simulink model "robotROSOmnidirectionalFBVisualizationV8_TrayectoriaV2"  (R2020a)
settings: Solver=FixedStepDiscrete  StartTime=0.0  StopTime=inf  FixedStep=0.01  RelTol=1e-3  EnableMultiTasking=on
undefined symbols (not defined in the file): Angular, Linear
libraries: robotlib x4
settings Model: Creator=The MathWorks, Inc.  LastModifiedBy=OsEmm
settings DataIOCC: LimitDataPoints=on  SaveFormat=Array  ReturnWorkspaceOutputs=off
settings OptimizationCC: LifeSpan=Inf  MaxStackSize=64
settings DebuggingCC: SolverPrmCheckMsg=warning  SFUnexpectedBacktrackingDiag=warning  SFNoUnconditionalDefaultTransitionDiag=warning  SFExecutionAtInitializationDiag=none  ArithmeticOperatorsInVariantConditions=warning
settings HardwareCC: ProdBitPerPointer=32  ProdBitPerSizeT=32  ProdBitPerPtrDiffT=32  ProdLargestAtomicFloat=None  ProdIntDivRoundTo=Undefined  ProdEndianess=Unspecified  ProdWordSize=32  ProdHWDeviceType=Generic->Unspecified (assume 32-bit Generic)  UseEmbeddedCoderFeatures=off
settings ModelReferenceCC: PropagateSignalLabelsOutOfModel=off
settings SFSimCC: SimUseLocalCustomCode=off
settings RTWCC: SystemTargetFile=ert.tlc  HardwareBoard=Robot Operating System (ROS)  TLCOptions=-aInlineSetEventsForThisBaseRateFcn=TLC_FALSE -aSuppressMultiTaskScheduler=TLC_FALSE -aRateBasedStepFcn=0  TemplateMakefile=ert_default_tmf  RTWUseLocalCustomCode=off  Toolchain=Catkin  TargetLang=C++
settings CodeAppCC: StateflowObjectComments=on
settings ERTTargetCC: MultiwordLength=2048  ERTCustomFileBanners=off  SupportContinuousTime=on  SupportNonInlinedSFcns=on  RemoveResetFunc=off  SupportVariableSizeSignals=on  ModelStepFunctionPrototypeControlCompliant=off  ConvertIfToSwitch=off  SuppressUnreachableDefaultCases=off
settings ConfigComp: CovMetricSettings=dw  CovHtmlReporting=on  CovSaveCumulativeToWorkspaceVar=on  CovSaveSingleToWorkspaceVar=on  CovExternalEMLEnable=off  CovSFcnEnable=off

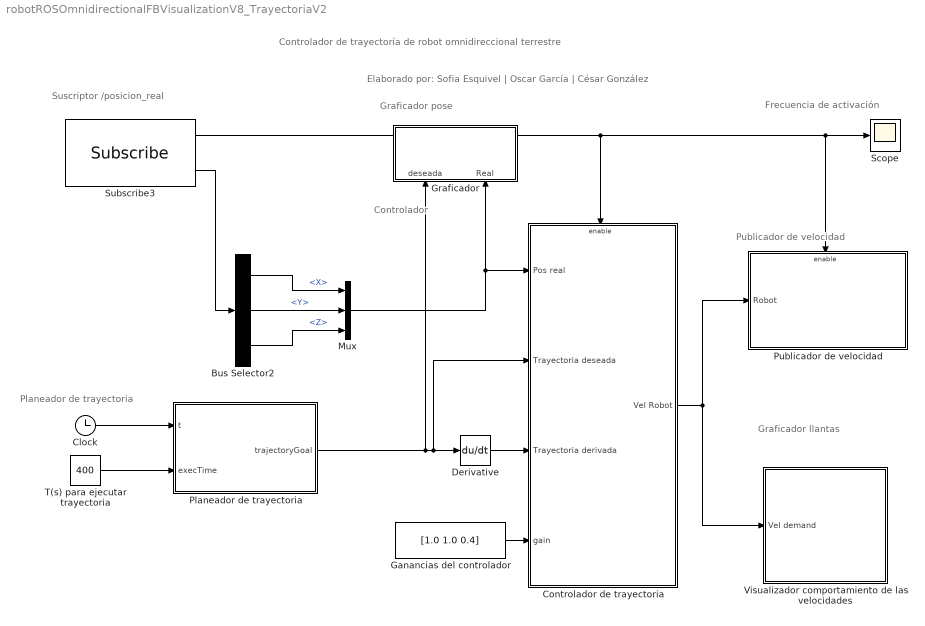
== system robotROSOmnidirectionalFBVisualizationV8_TrayectoriaV2 ==
  note: Frecuencia de activación
  note: Graficador llantas
  note: Publicador de velocidad
  note: Controlador
  note: Planeador de trayectoria
  note: Graficador pose
  note: Suscriptor /posicion_real
  note: Elaborado por: Sofia Esquivel | Oscar García | César González
  note: Controlador de trayectoría de robot omnidireccional terrestre
  Bus Selector2 : BusSelector  DialogController=Simulink.DDGSource_BusSelector  OutputSignals=Position.X,Position.Y,Position.Z
  Clock : Clock
  "Controlador de trayectoria " : Subsystem
  Derivative : Derivative
  Ganancias del controlador : Constant  Value=[1.0 1.0 0.4]
  Graficador : Subsystem
      settings: PortSchema="{\"entries\":[{\"content\":{\"sides\":[{\"content\":{\"connectorIds\":[]},\"type\":\"ConnectorPlacement.EquallySpacedRectSide\",\"uuid\":\"ca5a2c3c-1c6a-4a59-81b5-e28a07e4aa01\"},{\"content\":{\"connectorIds\":[],\"side\":\"RIGHT\"},\"type\":\"ConnectorPlacement.EquallySpacedRectSide\",\"uuid\":\"c66d5d4f-c2ca-4972-b9ac-4479b8aa35e9\"},{\"content\":{\"connectorIds\":[],\"side\":\"TOP\"},\"type\":\"ConnectorPlacement.EquallySpacedRectSide\",\"uuid\":\"6ec84811-9ba3-4605-b969-ad2255866a28\"},{\"content\":{\"connectorIds\":[\"In1\",\"In2\"],\"side\":\"BOTTOM\"},\"type\":\"ConnectorPlacement.EquallySpacedRectSide\",\"uuid\":\"853aacb6-3c5a-4075-8dd4-dac3c2fac177\"}]},\"type\":\"ConnectorPlacement.EquallySpacedConnector\",\"uuid\":\"ad9aaa3d-d9b2-4c1e-8caf-17ebb9e3127a\"}],\"packageUris\":[\"http://schema.mathworks.com/mf0/Connector/19700101\"],\"version\":\"1.0\"}"
  Mux : Mux  Inputs=3
  Planeador de trayectoria : MATLAB Function  TreatAsAtomicUnit=on
  Publicador de velocidad : Subsystem
  Scope : Scope
  Subscribe3 : robotlib/Subscribe  topicSource=Select from ROS network  topic=/posicion_real  messageType=geometry_msgs/Pose  sampleTime=-1  messageQueueLength=51
  "T(s) para ejecutar trayectoria " : Constant  Value=400
  "Visualizador comportamiento de las velocidades " : Subsystem
  wires:
  Subscribe3/1 -> Publicador de velocidad/Enable, Scope/1, "Controlador de trayectoria "/Enable
  Subscribe3/2 -> Bus Selector2/1
  Bus Selector2/1 -> Mux/1  "<X>"
  Bus Selector2/2 -> Mux/2  "<Y>"
  Bus Selector2/3 -> Mux/3  "<Z>"
  Mux/1 -> Graficador/2(Real), "Controlador de trayectoria "/1(Pos real)
  "Controlador de trayectoria "/1(Vel Robot) -> "Visualizador comportamiento de las velocidades "/1(Vel demand), Publicador de velocidad/1(Robot)
  Derivative/1 -> "Controlador de trayectoria "/3("Trayectoria derivada ")
  Clock/1 -> Planeador de trayectoria/1(t)
  "T(s) para ejecutar trayectoria "/1 -> Planeador de trayectoria/2(execTime)
  Planeador de trayectoria/1(trajectoryGoal) -> Graficador/1(deseada), "Controlador de trayectoria "/2(Trayectoria deseada), Derivative/1
  Ganancias del controlador/1 -> "Controlador de trayectoria "/4(gain)

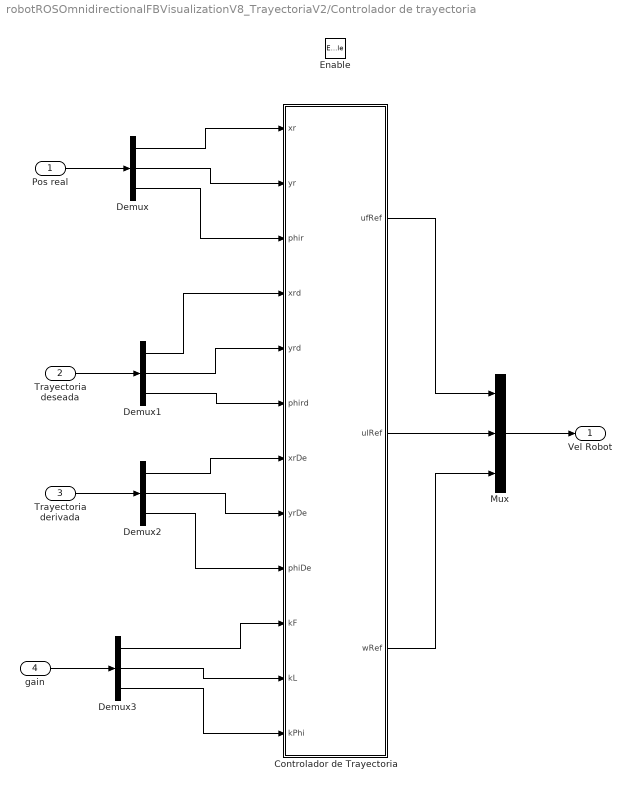
== system robotROSOmnidirectionalFBVisualizationV8_TrayectoriaV2/Controlador de trayectoria  ==
  Pos real : Inport
  Trayectoria deseada : Inport  Port=2
  "Trayectoria derivada " : Inport  Port=3
  gain : Inport  Port=4
  Enable : EnablePort
  Controlador de Trayectoria : MATLAB Function  TreatAsAtomicUnit=on
  Demux{,1..3} (4 alike) : Demux  Outputs=3
  Mux : Mux  Inputs=3
  Vel Robot : Outport
  wires:
  Pos real/1 -> Demux/1
  Demux/1 -> Controlador de Trayectoria/1(xr)
  Demux/2 -> Controlador de Trayectoria/2(yr)
  Demux/3 -> Controlador de Trayectoria/3(phir)
  Trayectoria deseada/1 -> Demux1/1
  Demux1/2 -> Controlador de Trayectoria/5(yrd)
  Demux1/1 -> Controlador de Trayectoria/4(xrd)
  Demux1/3 -> Controlador de Trayectoria/6(phird)
  Mux/1 -> Vel Robot/1
  Controlador de Trayectoria/1(ufRef) -> Mux/1
  Controlador de Trayectoria/2(ulRef) -> Mux/2
  Controlador de Trayectoria/3(wRef) -> Mux/3
  Demux2/3 -> Controlador de Trayectoria/9(phiDe)
  Demux2/1 -> Controlador de Trayectoria/7(xrDe)
  Demux2/2 -> Controlador de Trayectoria/8(yrDe)
  "Trayectoria derivada "/1 -> Demux2/1
  gain/1 -> Demux3/1
  Demux3/2 -> Controlador de Trayectoria/11(kL)
  Demux3/1 -> Controlador de Trayectoria/10(kF)
  Demux3/3 -> Controlador de Trayectoria/12(kPhi)

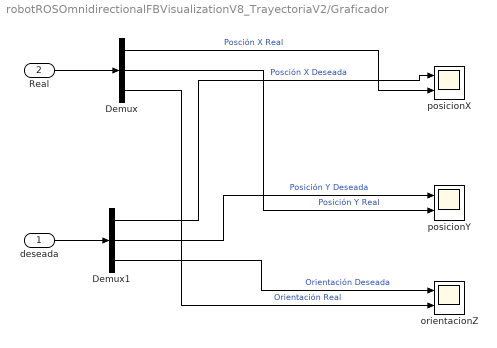
== system robotROSOmnidirectionalFBVisualizationV8_TrayectoriaV2/Graficador ==
  deseada : Inport
  Real : Inport  Port=2
  Demux : Demux  Outputs=3
  Demux1 : Demux  Outputs=3
  orientacionZ : Scope  NumInputPorts=2
  posicionX : Scope  NumInputPorts=2
  posicionY : Scope  NumInputPorts=2
  wires:
  Real/1 -> Demux/1
  deseada/1 -> Demux1/1
  Demux1/1 -> posicionX/1  "Posción X Deseada"
  Demux1/2 -> posicionY/1  "Posición Y Deseada"
  Demux1/3 -> orientacionZ/1  "Orientación Deseada"
  Demux/1 -> posicionX/2  "Posción X Real"
  Demux/2 -> posicionY/2  "Posición Y Real"
  Demux/3 -> orientacionZ/2  "Orientación Real"

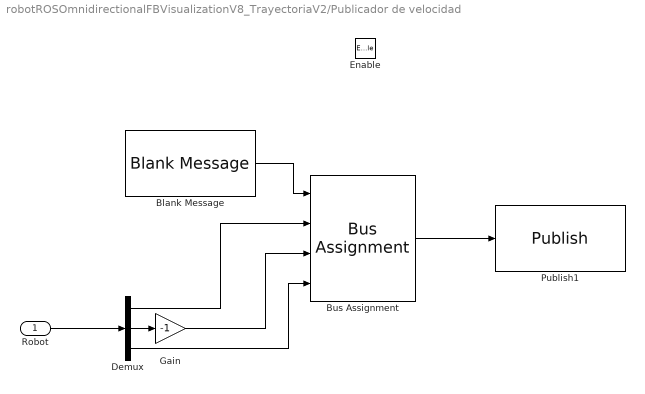
== system robotROSOmnidirectionalFBVisualizationV8_TrayectoriaV2/Publicador de velocidad ==
  Robot : Inport
  Enable : EnablePort
  Blank Message : robotlib/Blank Message  messageClass=Message  entityType=geometry_msgs/Twist  messageType=geometry_msgs/Twist  SampleTime=0.01
  Bus Assignment : BusAssignment  DialogController=Simulink.DDGSource_BusAssignment  AssignedSignals=Linear.X,Linear.Y,Angular.Z
  Demux : Demux  Outputs=3
  Gain : Gain  Gain=-1
  Publish1 : robotlib/Publish  topicSource=Select from ROS network  topic=/cmd_vel  messageType=geometry_msgs/Twist  messageQueueLength=105
  wires:
  Bus Assignment/1 -> Publish1/1
  Blank Message/1 -> Bus Assignment/1
  Robot/1 -> Demux/1
  Demux/2 -> Gain/1
  Demux/1 -> Bus Assignment/2
  Gain/1 -> Bus Assignment/3
  Demux/3 -> Bus Assignment/4

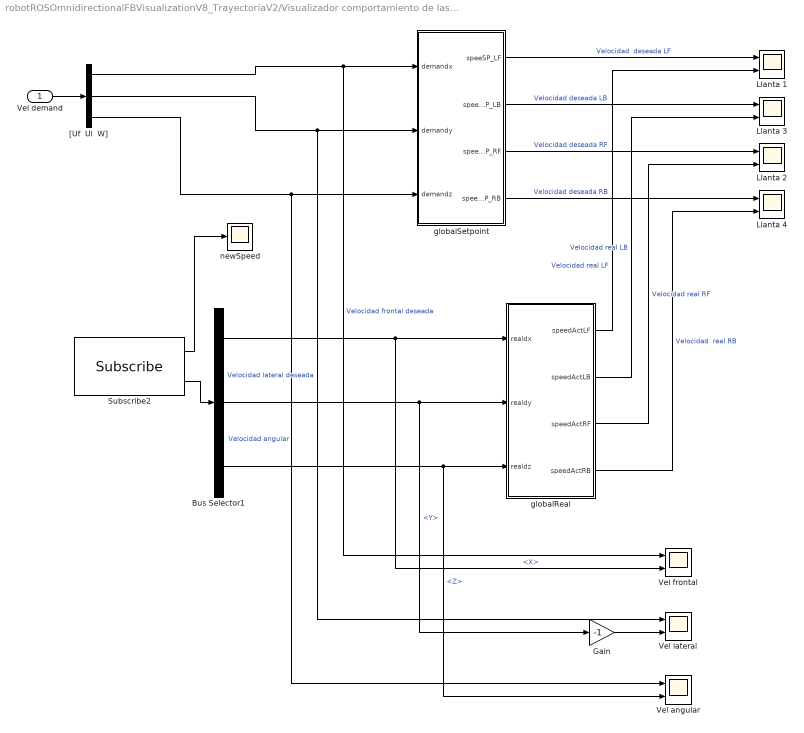
== system robotROSOmnidirectionalFBVisualizationV8_TrayectoriaV2/Visualizador comportamiento de las velocidades  ==
  Vel demand : Inport
  Bus Selector1 : BusSelector  DialogController=Simulink.DDGSource_BusSelector  OutputSignals=Vector_.X,Vector_.Y,Vector_.Z
  Gain : Gain  Gain=-1
  Llanta {1..4} (4 alike) : Scope  NumInputPorts=2
  Subscribe2 : robotlib/Subscribe  topicSource=Select from ROS network  topic=/speed  messageType=geometry_msgs/Vector3Stamped  sampleTime=-1  messageQueueLength=51
  Vel angular : Scope  NumInputPorts=2
  Vel frontal : Scope  NumInputPorts=2
  Vel lateral : Scope  NumInputPorts=2
  "[Uf  Ul  W]" : Demux  Outputs=3
  globalReal : MATLAB Function  TreatAsAtomicUnit=on
  globalSetpoint : MATLAB Function  TreatAsAtomicUnit=on
  newSpeed : Scope
  wires:
  Bus Selector1/2 -> globalReal/2(realdy), Gain/1  "<Y>"
  globalReal/3(speedActRF) -> Llanta 2/2  "Velocidad real RF"
  globalSetpoint/3(speedSP_RF) -> Llanta 2/1  "Velocidad deseada RF"
  Bus Selector1/1 -> globalReal/1(realdx), Vel frontal/2  "<X>"
  globalSetpoint/2(speedSP_LB) -> Llanta 3/1  "Velocidad deseada LB"
  globalReal/4(speedActRB) -> Llanta 4/2  "Velocidad  real RB"
  globalReal/2(speedActLB) -> Llanta 3/2  "Velocidad real LB"
  globalSetpoint/1(speeSP_LF) -> Llanta 1/1  "Velocidad  deseada LF"
  Subscribe2/2 -> Bus Selector1/1
  Bus Selector1/3 -> Vel angular/2, globalReal/3(realdz)  "<Z>"
  globalReal/1(speedActLF) -> Llanta 1/2  "Velocidad real LF"
  globalSetpoint/4(speedSP_RB) -> Llanta 4/1  "Velocidad deseada RB"
  "[Uf  Ul  W]"/1 -> Vel frontal/1, globalSetpoint/1(demandx)  "Velocidad frontal deseada"
  "[Uf  Ul  W]"/2 -> Vel lateral/1, globalSetpoint/2(demandy)  "Velocidad lateral deseada"
  "[Uf  Ul  W]"/3 -> Vel angular/1, globalSetpoint/3(demandz)  "Velocidad angular"
  Vel demand/1 -> "[Uf  Ul  W]"/1
  Subscribe2/1 -> newSpeed/1
  Gain/1 -> Vel lateral/2

== matlab function robotROSOmnidirectionalFBVisualizationV8_TrayectoriaV2/Visualizador comportamiento de las velocidades /globalReal ==
  data: realdx input; speedActLF output; realdy input; realdz input; speedActLB output; speedActRF output; speedActRB output
function [speedActLF, speedActLB, speedActRF, speedActRB] = robotToWheelSpeed(realdx, realdy, realdz)

    constR = 20;
    Lx = 0.192;
    Ly = 0.105;
    
    speedActLF = constR * (realdx - realdy -Lx*realdz - Ly* realdz);
    speedActRF = constR *(realdx + realdy + Lx*realdz + Ly*realdz);
    speedActLB = constR * (realdx + realdy -Lx*realdz - Ly*realdz);
    speedActRB = constR * (realdx -realdy + Lx*realdz + Ly*realdz);

== matlab function robotROSOmnidirectionalFBVisualizationV8_TrayectoriaV2/Controlador de trayectoria /Controlador de Trayectoria ==
  data: xr input; yr input; phir input; xrd input; yrd input; phird input; ufRef output; ulRef output; wRef output; xrDe input; yrDe input; phiDe input; kF input; kL input; kPhi input
function [ufRef, ulRef, wRef] = fcn(xr, yr ,phir, xrd, yrd, phird, xrDe, yrDe, phiDe, kF, kL, kPhi)

%%%%%%%%%%%%%%%%%%% Controller %%%%%%%%%%%%%%%%%%%%%%%%%
% % 
% %         xrd = 1;
% %         yrd = 1;
% %     a) error
% %    
        xre = xrd - xr;  % error positon (x axis) in meters (m)
        yre = yrd - yr;  % error positon (y axis) in meters (m)
        phire = phird - phir; 
% % %         xre = eInput(1);
% % %         yre = eInput(2);
% % %         phire = 0;
        he = [xre yre phire]'; % error vector
  
    % b) Jacobian Matrix
        J11 = cos(phir);
        J12 = -sin(phir);
        J13 = 0;

        J21 = sin(phir);
        J22 = cos(phir);
        J23 = 0;
        
        J31 = 0;
        J32 = 0;
        J33 = 1;

        J=[J11 J12 J13;...
           J21 J22 J23;...
           J31 J32 J33];

%    % c) Control parameters
%         K = [0.2    0    0;...
%              0    0.3    0;...
%              0      0    0.1];
         

         % c) Control parameters
        K = [kF    0    0;...
             0    kL    0;...
             0      0    kPhi];
         
        hdp = [xrDe yrDe phiDe]';
    
   % d) Law control
        %qpref = pinv(J)*(K*he);
        %qpref = pinv(J)*(K*tanh(he));
        
        %qpref = pinv(J)*(hdp+K*he);
        qpref = pinv(J)*(hdp+K*tanh(he));
        
   % e) Separate action control
        ufRef = qpref(1);
        ulRef = qpref(2);
        wRef  = qpref(3);

== matlab function robotROSOmnidirectionalFBVisualizationV8_TrayectoriaV2/Planeador de trayectoria ==
  data: trajectoryGoal output; t input; execTime input
function trajectoryGoal  = fcn(t, execTime)

% [trajectoryGoal, trajectoryDerived] = fcn(t, execTime)


       
% % % % % % 
% % % % % % 
% % % % % %         xGoal=0.5*cos(0.1*t);
% % % % % %         yGoal=0.5*sin(0.1*t);
% % % % % %         phiGoal = 0;
% % % % % % 
% % % % % %         xGoald = 1*0.3*cos(0.3*t);
% % % % % %         yGoald = -1*0.3*sin(0.3*t);
% % % % % %         phiGoald =  0;
% % % % % %    

% wx=1*sin(0.3*t);
% wy=1*cos(0.3*t);
% wz = (pi/180)*90;
% 
% % hxdp=1*0.3*cos(0.3*t);
% % hydp=-1*0.3*sin(0.3*t);
% % phidp =  0*zeros(1,Q);
% 
%  trajectoryGoal = [wx wy wz];
% 

% % 
% % pointNumber = size(trajPoints); 
% %     
% %     n = pointNumber(1);
% %     
% %     i = 1; 
% %     for i: i++: i < n
% %         tf[i] = (i * ttotal)/n; 
% %         
% %     end 
% %     
% % 
% %     traySection = 1;     
% %     if t <= tf(traySection)
% %         
% %         a2x = (3/tf(traySection)^2)*( P(traySection++, 1) - P(traySection, 1) );
% %         a3x = (-2/tf(traySection^3)*( P(traySection++, 1) - P(traySection, 1) );
% % 
% %         a2y = (3/tf1^2)*(P2(2)-P1(2));
% %         a3y = (-2/tf1^3)*(P2(2)-P1(2));
% % 
% %         wx = P1(1) + a2x*(t^2) +  a3x*(t^3);
% %         wy = P1(2) + a2y*(t^2) +  a3y*(t^3);
% %         
% %         wxd = 2*a2x*t + 3*a3x*(t^2);
% %         wyd = 2*a2y*t + 3*a3y*(t^2);
% % 
% %         
% %     elseif t > tf(traySection) && t <= tf(traySection++)
% %         
% %         
% % 
% % 





% % % % % % % % 
% % % % % % % %     ttotal = execTime;  n = 4;
% % % % % % % %     
% % % % % % % %     
% % % % % % % %     tf1 = ttotal/n;     P1 = 0.66*[1 , 1]; 
% % % % % % % %     tf2 = 2*ttotal/n;   P2 = 0.66*[3 , 1];     
% % % % % % % %     tf3 = 3*ttotal/n;   P3 = 0.66*[3 , 3];
% % % % % % % %     tf4 = 4*ttotal/n;   P4 = 0.66*[1 , 3];    
% % % % % % % %     
% % % % % % % %     wz = 5*pi/180;
% % % % % % % % %     wzd = 0;
% % % % % % % % 
% % % % % % % %     if t <= tf1       
% % % % % % % % 
% % % % % % % %         a2x = (3/tf1^2)*(P2(1)-P1(1));
% % % % % % % %         a3x = (-2/tf1^3)*(P2(1)-P1(1));
% % % % % % % % 
% % % % % % % %         a2y = (3/tf1^2)*(P2(2)-P1(2));
% % % % % % % %         a3y = (-2/tf1^3)*(P2(2)-P1(2));
% % % % % % % % 
% % % % % % % %         wx = P1(1) + a2x*(t^2) +  a3x*(t^3);
% % % % % % % %         wy = P1(2) + a2y*(t^2) +  a3y*(t^3);
% % % % % % % %         
% % % % % % % % %         wxd = 2*a2x*t + 3*a3x*(t^2);
% % % % % % % % %         wyd = 2*a2y*t + 3*a3y*(t^2);
% % % % % % % %     
% % % % % % % %         
% % % % % % % %     
% % % % % % % % 
% % % % % % % %     elseif (t > tf1 && t <= tf2)
% % % % % % % % 
% % % % % % % %         a2x = (3/tf2^2)*(P3(1)-P2(1));
% % % % % % % %         a3x = (-2/tf2^3)*(P3(1)-P2(1));
% % % % % % % % 
% % % % % % % %         a2y = (3/tf2^2)*(P3(2)-P2(2));
% % % % % % % %         a3y = (-2/tf2^3)*(P3(2)-P2(2));
% % % % % % % % 
% % % % % % % %         wx = P2(1) + a2x*(t^2) +  a3x*(t^3);
% % % % % % % %         wy = P2(2) + a2y*(t^2) +  a3y*(t^3);
% % % % % % % %         
% % % % % % % % %         wxd = 2*a2x*t + 3*a3x*(t^2);
% % % % % % % % %         wyd = 2*a2y*t + 3*a3y*(t^2);
% % % % % % % % 
% % % % % % % %     
% % % % % % % %     
% % % % % % % % 
% % % % % % % %     elseif (t > tf2 && t <= tf3)
% % % % % % % % 
% % % % % % % %         a2x = (3/tf3^2)*(P4(1)-P3(1));
% % % % % % % %         a3x = (-2/tf3^3)*(P4(1)-P3(1));
% % % % % % % % 
% % % % % % % %         a2y = (3/tf3^2)*(P4(2)-P3(2));
% % % % % % % %         a3y = (-2/tf3^3)*(P4(2)-P3(2));
% % % % % % % % 
% % % % % % % %         wx = P3(1) + a2x*(t^2) +  a3x*(t^3);
% % % % % % % %         wy = P3(2) + a2y*(t^2) +  a3y*(t^3);
% % % % % % % %         
% % % % % % % % %         wxd = 2*a2x*t + 3*a3x*(t^2);
% % % % % % % % %         wyd = 2*a2y*t + 3*a3y*(t^2);
% % % % % % % %     
% % % % % % % % 
% % % % % % % %     elseif (t > tf3 && t <= tf4)
% % % % % % % % 
% % % % % % % %         a2x = (3/tf4^2)*(P1(1)-P4(1));
% % % % % % % %         a3x = (-2/tf4^3)*(P1(1)-P4(1));
% % % % % % % % 
% % % % % % % %         a2y = (3/tf4^2)*(P1(2)-P4(2));
% % % % % % % %         a3y = (-2/tf4^3)*(P1(2)-P4(2));
% % % % % % % % 
% % % % % % % %         wx = P4(1) + a2x*(t^2) +  a3x*(t^3);
% % % % % % % %         wy = P4(2) + a2y*(t^2) +  a3y*(t^3);
% % % % % % % %         
% % % % % % % % %         wxd = 2*a2x*t + 3*a3x*(t^2);
% % % % % % % % %         wyd = 2*a2y*t + 3*a3y*(t^2);
% % % % % % % % %     
% % % % % % % %    
% % % % % % % %     else   
% % % % % % % %         
% % % % % % % %         wx = 0;
% % % % % % % %         wy = 0;
% % % % % % % %     end
% % % % % % % %                                                               
% % % % % % % %                                                  
% % % % % % % %     trajectoryGoal = [wx wy wz];
   
%     trajectoryDerived = [wxd wyd wzd];
    


%         xrd = -3;  % desired position (x axis) in meters (m)
%         yrd = 3;  % desired position (y axis) in meters (m)
%         phird = 0; 
% % %    
% %     elseif (opc == 1)
% %         %Trayectoria deseada 
% %         T = 40;     b =2*pi/T;
% %         Pd = [cos(b*t); sin(b*t)];
% %         dPd = [-b*sin(b*t); b*cos(b*t)];
% % 
% %         
% %     else 


    ttotal = execTime;  n = 4;
    
    
    tf1 = ttotal/n;     P1 = 0.66*[1 , 1]; 
    tf2 = 2*ttotal/n;   P2 = 0.66*[3 , 1];     
    tf3 = 3*ttotal/n;   P3 = 0.66*[3 , 3];
    tf4 = 4*ttotal/n;   P4 = 0.66*[1 , 3];    
    
    
%     wzd = 0;

    if t <= tf1       

        tfe = tf1; ti = 0;
        x0 = P1(1);    xf = P2(1);
        y0 = P1(2);    yf = P2(2);
        
    

    elseif (t > tf1 && t <= tf2)

   
        tfe = tf2 - tf1; ti = tf1;
        x0 = P2(1);    xf = P3(1);
        y0 = P2(2);    yf = P3(2);
    

    elseif (t > tf2 && t <= tf3)

        tfe = tf3 - tf2; ti = tf2;
        x0 = P3(1);    xf = P4(1);
        y0 = P3(2);    yf = P4(2);


    elseif (t > tf3 && t <= tf4)

         tfe = tf4 - tf3; ti = tf3;
        x0 = P4(1);    xf = P1(1);
        y0 = P4(2);    yf = P1(2);

    else   
        
        tfe = 0; ti = tf4;
        x0 = P1(1);    xf = P1(1);
        y0 = P1(2);    yf = P1(2);
    end
    
     A = [   tfe^3,    tfe^4,    tfe^5,    tfe^6,      tfe^7;
         3*tfe^2,  4*tfe^3,  5*tfe^4,  6*tfe^5,    7*tfe^6;
           6*tfe, 12*tfe^2, 20*tfe^3,  30*tfe^4,  42*tfe^5;
               6,   24*tfe, 60*tfe^2, 120*tfe^3, 210*tfe^4;
               0,       24,  120*tfe, 360*tfe^2, 840*tfe^3]; 
   
   X = [xf-x0; 0; 0; 0; 0]; 
   Y = [yf-y0; 0; 0; 0; 0]; 
   
   
   bx = A\X;  %inv(A)*X
   by = A\Y;
   
   a3x=bx(1,1);     a4x=bx(2,1);    a5x=bx(3,1); a6x=bx(4,1); a7x=bx(5,1);
   a3y=by(1,1);     a4y=by(2,1);    a5y=by(3,1); a6y=by(4,1); a7y=by(5,1);
    
   ta = t - ti; %se actualiza el tiempo para que siempre vaya de 0 a 10
   
   wx = x0 + a3x*(ta^3) + a4x*(ta^4) + a5x*(ta^5) + a6x*(ta^6) + a7x*(ta^7);
   wy = y0 + a3y*(ta^3) + a4y*(ta^4) + a5y*(ta^5) + a6y*(ta^6) + a7y*(ta^7);

   wz = (pi/180)*90;
                                                
                                        
    trajectoryGoal = [wx wy wz];
    

end

== matlab function robotROSOmnidirectionalFBVisualizationV8_TrayectoriaV2/Visualizador comportamiento de las velocidades /globalSetpoint ==
  data: demandx input; speeSP_LF output; demandy input; demandz input; speedSP_LB output; speedSP_RF output; speedSP_RB output
function [speeSP_LF, speedSP_LB, speedSP_RF, speedSP_RB] = robotToWheelSpeedSetPoint(demandx, demandy, demandz)

    constR = 20;
    Lx = 0.192;
    Ly = 0.105;
    
    speeSP_LF = constR * (demandx - demandy -Lx*demandz - Ly* demandz);
    speedSP_RF = constR *(demandx + demandy + Lx*demandz + Ly*demandz);
    speedSP_LB = constR * (demandx + demandy -Lx*demandz - Ly*demandz);
    speedSP_RB = constR * (demandx -demandy + Lx*demandz + Ly*demandz);
